simulink model "MM1K"  (R2020b)
settings: Solver=VariableStepDiscrete  StartTime=0.0  StopTime=stopTime  FixedStep=0.01  RelTol=1e-3
values from neighbouring files (symbols this model uses):
  capacity = Simulink.Parameter    [mm1k.m]    (also in server_report.m)
  n = [1:C]    [pdfMM1K.m]
undefined symbols (not defined in the file or in its folder): m
libraries: simulink x1
settings Model: Creator=pcuijper  LastModifiedBy=Ander
settings SolverCC: ZeroCrossControl=DisableAll
settings DataIOCC: ReturnWorkspaceOutputs=off
settings DebuggingCC: ArithmeticOperatorsInVariantConditions=warning
settings SFSimCC: SimUseLocalCustomCode=off  CustomCodeUndefinedFunction=UseInterfaceOnly
settings RTWCC: RTWUseLocalCustomCode=off
settings CodeAppCC: StateflowObjectComments=on

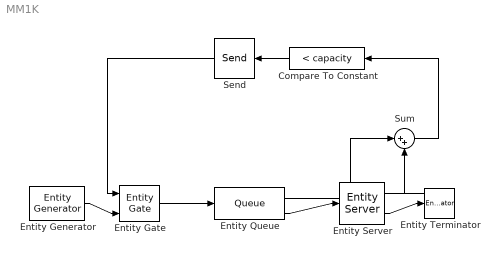
== system MM1K ==
  Compare To Constant : simulink/Logic and Bit Operations/Compare To Constant  relop=<  const=capacity  OutDataTypeStr=uint8
  Entity Gate : EntityGate  InputPortMessageModes=m,m  OutputPortMessageModes=m  OpenGateAtSimulationStart=on
  Entity Generator : EntityGenerator  OutputPortMessageModes=m  TimeSource=MATLAB action  IntergenerationTimeAction=|  GenerateEntityAtSimulationStart=off  EntityType=Structured  EntityTypeName=Entity
      | persistent rngInit;
      | 
      | if isempty(rngInit)
      |     seed = mySeed;
      |     rng(seed);
      |     rngInit = true;
      | end
      | 
      | dt = -interArrivalTime * log(1 - rand());
  Entity Queue : Queue  InputPortMessageModes=m  OutputPortMessageModes=n,m  Capacity=capacity  NumberEntitiesInBlock=on
      settings: OutputPortMap=o1,o5
  Entity Server : EntityServer  InputPortMessageModes=m  OutputPortMessageModes=n,m  Capacity=1  ServiceTimeSource=MATLAB action  ServiceTimeValue=rand(1,1)  ServiceTimeAction=|  NumberEntitiesInBlock=on
      | persistent rngInit;
      | 
      | if isempty(rngInit)
      |     seed = mySeed+1;
      |     rng(seed);
      |     rngInit = true;
      | end
      | 
      | dt = -interServiceTime * log(1 - rand());
      settings: OutputPortMap=o1,o9
  Entity Terminator : EntityTerminator  InputPortMessageModes=m
  Send : Send  OutputPortMessageModes=m
  Sum : Sum  Inputs=|++
  wires:
  Entity Generator/1 -> Entity Gate/2
  Entity Queue/2 -> Entity Server/1
  Entity Server/2 -> Entity Terminator/1
  Entity Server/1 -> Sum/2
  Entity Queue/1 -> Sum/1
  Compare To Constant/1 -> Send/1
  Entity Gate/1 -> Entity Queue/1
  Send/1 -> Entity Gate/1
  Sum/1 -> Compare To Constant/1
